simulink model "chap07_07_07_mdl"  (R2013b)
settings: Solver=ode45  StartTime=0.0  StopTime=10.0  RelTol=1e-3
settings Model: Creator=Administrator  LastModifiedBy=sunzx.fnst

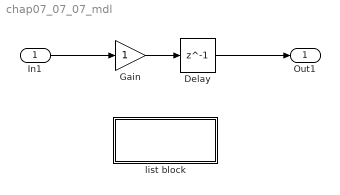
== system chap07_07_07_mdl ==
  In1 : Inport
  Delay : Delay  DelayLength=1  InitialCondition=0  SampleTime=1
  Gain : Gain
  list block : Subsystem  mask(Hyo_Custom){g_enable=on, g_list=list block}
      mask prompts: g_enable "List blocks"; g_list "Block list"
      mask help: This block can supply a list of all blocks in this model if user checks on the "list blocks" check-box.
      mask init:
      | set_param(gcbh, 'MaskSelfModifiable' , 'off');
      mask Callback g_enable: listblock_callback('g_enable');
      mask TypeOptions g_list: In1 | Delay | Gain | list block | Out1
      mask Callback g_list: listblock_callback('g_list');
      mask Display: disp('List Blocks');
  Out1 : Outport
  wires:
  In1/1 -> Gain/1
  Delay/1 -> Out1/1
  Gain/1 -> Delay/1

== system chap07_07_07_mdl/list block ==
